simulink model "main"  (R2024a)
settings: Solver=VariableStepAuto  StartTime=0.0  StopTime=1  MaxStep=1e-4  RelTol=1e-3
InitFcn:
  | parametros
values from neighbouring files (symbols this model uses):
  alpha_cu = 3.9 *10^-3    (= 0.0039)    [parametros.m]
  b_l = 0.1    [parametros.m]
  b_m = 1.5 * 10^-5    (= 1.5e-05)    [parametros.m]
  C_ts = 0.818    [parametros.m]
  J_l = (m*l_cm^2 + J_cm) + (m_l * l_l^2)    (= 0.0833)    [parametros.m]
  J_m = 1.4 * 10^-5    (= 1.4e-05)    [parametros.m]
  k_l = m * g * l_cm + m_l * g * l_l    (= 2.4516625)    [parametros.m]
  L_d = 6.6 * 10^-3    (= 0.0066)    [parametros.m]
  L_ls = 0.8 * 10^-3    (= 0.0008)    [parametros.m]
  L_q = 5.8 * 10^-3    (= 0.0058)    [parametros.m]
  lambda_m = 0.016    [parametros.m]
  P_p = 3    [parametros.m]
  r = 120    [parametros.m]
  R_s_40 = 1.02    [parametros.m]
  R_ts_amb = 146.7    [parametros.m]
  Temp_s_ref = 40    [parametros.m]
(part 1 of 3)
settings Model: Creator=Usuario  LastModifiedBy=Usuario
settings RTWCC: GPUComputeCapability=3.5

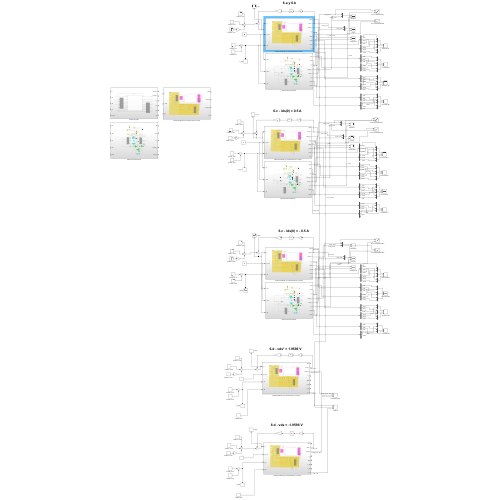
[thumbnail: Simulink's stored preview of the top-level diagram]
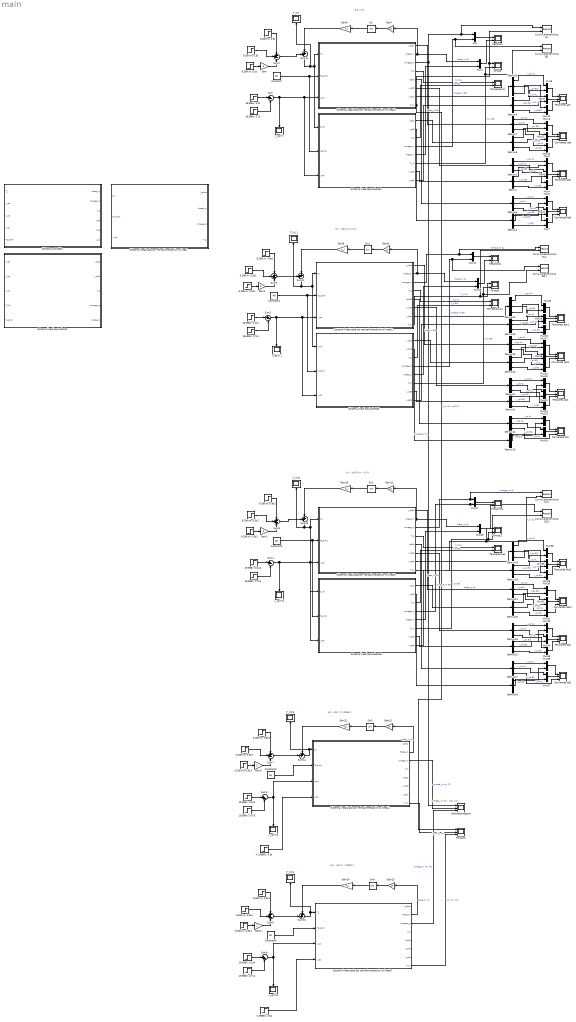
== system main ==
  note: omega_m NL - vds = 0
  note: 6.a y 6.b
  note: 6.c - ids(0) = 0.5 A
  note: 6.c - ids(0) = - 0.5 A
  note: 6.d - vds = -1.9596 V
  note: 6.d - vds* = 1.9596 V
  "+1.9596V, 0.5s" : Step  Time=.5  After=1.9596  SampleTime=0
  "-1.9596V, 0.5s" : Step  Time=.5  After=-1.9596  SampleTime=0
  19.596V, 0.1s{,1..4} (5 alike) : Step  Time=.1  After=19.596  SampleTime=0
  19.596V, 0.7s{,1..4} (5 alike) : Step  Time=.7  After=19.596  SampleTime=0
  6.28N.m, 0.3s{,1..4} (5 alike) : Step  Time=0.3  After=6.28  SampleTime=0
  6.28N.m, 0.5s{,1..4} (5 alike) : Step  Time=.5  After=6.28  SampleTime=0
  6.28N.m, 0.9s{,1..4} (5 alike) : Step  Time=.9  After=6.28  SampleTime=0
  Constant{,1..4} (5 alike) : Constant  Value=40
  Corrientes abc : Scope  NumInputPorts=3
  Corrientes abc1 : Scope  NumInputPorts=3
  Corrientes abc2 : Scope  NumInputPorts=3
  Corrientes qd0 : Scope  NumInputPorts=3
  Corrientes qd1 : Scope  NumInputPorts=3
  Corrientes qd2 : Scope  NumInputPorts=3
  Curva característica EQ : Record  FileSettingsInternal="{\"entries\":[{\"content\":{\"excelSettings\":{\"content\":{},\"type\":\"Streamout.ExcelSettings\"}},\"type\":\"Streamout.FileSettingStorage\",\"uuid\":\"\"}],\"packageUris\":[\"http:\\/\\/schema.mathworks.com\\/mf0\\/streamout_blocks\\/R2020a\"],\"version\":\"1.0\"}"  Layout=[1 1]  SignalsInternal="{\"entries\":[{\"content\":{},\"type\":\"RecordBlkView.InputSignals\",\"uuid\":\"\"}],\"packageUris\":[\"http:\\/\\/schema.mathworks.com\\/mf0\\/streamout_blocks\\/R2020a\"],\"version\":\"1.0\"}"  VisualizationBindings="{\"xyplotplugin\":{\"info\":[{\"series\":[{\"bindingParametersList\":[{\"parameter\":\"X-Axis\",\"signalID\":24,\"signalName\":\"omega_m EQ\"},{\"parameter\":\"Y-Axis\",\"signalID\":27,\"signalName\":\"T_m EQ\"}],\"seriesID\":0}],\"subplotID\":1}]}}"  CompatibilityTag=XY
  Curva característica EQ1 : Record  FileSettingsInternal="{\"entries\":[{\"content\":{\"excelSettings\":{\"content\":{},\"type\":\"Streamout.ExcelSettings\"}},\"type\":\"Streamout.FileSettingStorage\",\"uuid\":\"\"}],\"packageUris\":[\"http:\\/\\/schema.mathworks.com\\/mf0\\/streamout_blocks\\/R2020a\"],\"version\":\"1.0\"}"  Layout=[1 1]  SignalsInternal="{\"entries\":[{\"content\":{},\"type\":\"RecordBlkView.InputSignals\",\"uuid\":\"\"}],\"packageUris\":[\"http:\\/\\/schema.mathworks.com\\/mf0\\/streamout_blocks\\/R2020a\"],\"version\":\"1.0\"}"  VisualizationBindings="{\"xyplotplugin\":{\"info\":[{\"series\":[{\"bindingParametersList\":[{\"parameter\":\"X-Axis\",\"signalID\":40,\"signalName\":\"omega_m EQ\"},{\"parameter\":\"Y-Axis\",\"signalID\":43,\"signalName\":\"T_m EQ\"}],\"seriesID\":0}],\"subplotID\":1}]}}"  CompatibilityTag=XY
  Curva característica EQ2 : Record  FileSettingsInternal="{\"entries\":[{\"content\":{\"excelSettings\":{\"content\":{},\"type\":\"Streamout.ExcelSettings\"}},\"type\":\"Streamout.FileSettingStorage\",\"uuid\":\"\"}],\"packageUris\":[\"http:\\/\\/schema.mathworks.com\\/mf0\\/streamout_blocks\\/R2020a\"],\"version\":\"1.0\"}"  Layout=[1 1]  SignalsInternal="{\"entries\":[{\"content\":{},\"type\":\"RecordBlkView.InputSignals\",\"uuid\":\"\"}],\"packageUris\":[\"http:\\/\\/schema.mathworks.com\\/mf0\\/streamout_blocks\\/R2020a\"],\"version\":\"1.0\"}"  VisualizationBindings="{\"xyplotplugin\":{\"info\":[{\"series\":[{\"bindingParametersList\":[{\"parameter\":\"X-Axis\",\"signalID\":48,\"signalName\":\"omega_m EQ\"},{\"parameter\":\"Y-Axis\",\"signalID\":51,\"signalName\":\"T_m EQ\"}],\"seriesID\":0}],\"subplotID\":1}]}}"  CompatibilityTag=XY
  Curva característica NL : Record  FileSettingsInternal="{\"entries\":[{\"content\":{\"excelSettings\":{\"content\":{},\"type\":\"Streamout.ExcelSettings\"}},\"type\":\"Streamout.FileSettingStorage\",\"uuid\":\"\"}],\"packageUris\":[\"http:\\/\\/schema.mathworks.com\\/mf0\\/streamout_blocks\\/R2020a\"],\"version\":\"1.0\"}"  Layout=[1 1]  SignalsInternal="{\"entries\":[{\"content\":{},\"type\":\"RecordBlkView.InputSignals\",\"uuid\":\"\"}],\"packageUris\":[\"http:\\/\\/schema.mathworks.com\\/mf0\\/streamout_blocks\\/R2020a\"],\"version\":\"1.0\"}"  VisualizationBindings="{\"xyplotplugin\":{\"info\":[{\"series\":[{\"bindingParametersList\":[{\"parameter\":\"X-Axis\",\"signalID\":32,\"signalName\":\"omega_m NL\"},{\"parameter\":\"Y-Axis\",\"signalID\":35,\"signalName\":\"T_m NL - Vds= 0\"}],\"seriesID\":0}],\"subplotID\":1}]}}"  CompatibilityTag=XY
  Curva característica NL1 : Record  FileSettingsInternal="{\"entries\":[{\"content\":{\"excelSettings\":{\"content\":{},\"type\":\"Streamout.ExcelSettings\"}},\"type\":\"Streamout.FileSettingStorage\",\"uuid\":\"\"}],\"packageUris\":[\"http:\\/\\/schema.mathworks.com\\/mf0\\/streamout_blocks\\/R2020a\"],\"version\":\"1.0\"}"  Layout=[1 1]  SignalsInternal="{\"entries\":[{\"content\":{},\"type\":\"RecordBlkView.InputSignals\",\"uuid\":\"\"}],\"packageUris\":[\"http:\\/\\/schema.mathworks.com\\/mf0\\/streamout_blocks\\/R2020a\"],\"version\":\"1.0\"}"  VisualizationBindings="{\"xyplotplugin\":{\"info\":[{\"series\":[{\"bindingParametersList\":[{\"parameter\":\"X-Axis\",\"signalID\":16,\"signalName\":\"omega_m NL\"},{\"parameter\":\"Y-Axis\",\"signalID\":19,\"signalName\":\"T_m NL\"}],\"seriesID\":0}],\"subplotID\":1}]}}"  CompatibilityTag=XY
  Curva característica NL2 : Record  FileSettingsInternal="{\"entries\":[{\"content\":{\"excelSettings\":{\"content\":{},\"type\":\"Streamout.ExcelSettings\"}},\"type\":\"Streamout.FileSettingStorage\",\"uuid\":\"\"}],\"packageUris\":[\"http:\\/\\/schema.mathworks.com\\/mf0\\/streamout_blocks\\/R2020a\"],\"version\":\"1.0\"}"  Layout=[1 1]  SignalsInternal="{\"entries\":[{\"content\":{},\"type\":\"RecordBlkView.InputSignals\",\"uuid\":\"\"}],\"packageUris\":[\"http:\\/\\/schema.mathworks.com\\/mf0\\/streamout_blocks\\/R2020a\"],\"version\":\"1.0\"}"  VisualizationBindings="{\"xyplotplugin\":{\"info\":[{\"series\":[{\"bindingParametersList\":[{\"parameter\":\"X-Axis\",\"signalID\":8,\"signalName\":\"omega_m NL\"},{\"parameter\":\"Y-Axis\",\"signalID\":11,\"signalName\":\"T_m NL\"}],\"seriesID\":0}],\"subplotID\":1}]}}"  CompatibilityTag=XY
  Demux{,1..23} (24 alike) : Demux  Outputs=3
  Gain{,1..4} (5 alike) : Gain  Gain=2
  Gain{6,8,10,12,14} (5 alike) : Gain  Gain=k_l
  Gain{7,9,11,13,15} (5 alike) : Gain  Gain=1/r
  Mecánico : Scope  NumInputPorts=2
  Mecánico1 : Scope  NumInputPorts=2
  Mecánico2 : Scope  NumInputPorts=2
  Mux{,1..39} (40 alike) : Mux  Inputs=2
  Sin{,1..4} (5 alike) : Trigonometry
  Sistema completo : Subsystem
  Sistema lineal equivalente : Subsystem
  Sistema lineal equivalente1 : Subsystem
  Sistema lineal equivalente2 : Subsystem
  Sistema lineal equivalente3 : Subsystem
  Sistema linealizado por retroalimentación no lineal : Subsystem
  Sistema linealizado por retroalimentación no lineal1 : Subsystem
  Sistema linealizado por retroalimentación no lineal2 : Subsystem
  Sistema linealizado por retroalimentación no lineal3 : Subsystem
  Sistema linealizado por retroalimentación no lineal4 : Subsystem
  Sistema linealizado por retroalimentación no lineal5 : Subsystem
  Sum{,2,4,6,8} (5 alike) : Sum  Inputs=|+-
  Sum{1,3,5,7,9} (5 alike) : Sum  Inputs=++-
  Sum{11..15} (5 alike) : Sum  Inputs=++|
  T_l(t){,1..4} (5 alike) : Scope
  Temperatura : Scope  NumInputPorts=2
  Temperatura1 : Scope  NumInputPorts=2
  Temperatura2 : Scope  NumInputPorts=2
  Tensiones abc : Scope  NumInputPorts=3
  Tensiones abc1 : Scope  NumInputPorts=3
  Tensiones abc2 : Scope  NumInputPorts=3
  Tensiones qd0 : Scope  NumInputPorts=3
  Tensiones qd1 : Scope  NumInputPorts=3
  Tensiones qd2 : Scope  NumInputPorts=3
  Torque : Scope  NumInputPorts=2
  Torque 5 : Scope  NumInputPorts=3
  Torque1 : Scope  NumInputPorts=2
  Torque2 : Scope  NumInputPorts=2
  Velocidad angular : Scope  NumInputPorts=3
  v_qs(t){,1..4} (5 alike) : Scope
  wires:
  Sistema linealizado por retroalimentación no lineal1/2(theta_m) -> Gain7/1, Mux1/1  "theta_m NL"
  Sistema linealizado por retroalimentación no lineal1/3(omega_m) -> Velocidad angular/1, Curva característica NL/1, Mux/1  "omega_m NL"
  Sistema lineal equivalente1/5(theta_m) -> Mux1/2  "theta_m EQ"
  Sistema lineal equivalente1/4(omega_m) -> Curva característica EQ/1, Mux/2  "omega_m EQ"
  "19.596V, 0.1s"/1 -> Sum/1
  "19.596V, 0.7s"/1 -> Sum/2
  Sum/1 -> Sistema lineal equivalente1/3(v_qs), Sistema linealizado por retroalimentación no lineal1/3(v_qs), v_qs(t)/1
  "6.28N.m, 0.5s"/1 -> Gain/1
  Gain/1 -> Sum1/3
  "6.28N.m, 0.3s"/1 -> Sum1/2
  "6.28N.m, 0.9s"/1 -> Sum1/1
  Sum1/1 -> Sum11/1
  Constant/1 -> Sistema lineal equivalente1/2(T_amb), Sistema linealizado por retroalimentación no lineal1/2(Tº_amb)
  Mux/1 -> Mecánico/1
  Mux1/1 -> Mecánico/2
  Sistema lineal equivalente1/6(T_m) -> Curva característica EQ/2, Torque/2  "T_m EQ"
  Sistema lineal equivalente1/3(T_s) -> Temperatura/2  "T_s EQ"
  Sistema linealizado por retroalimentación no lineal1/4(T_s) -> Temperatura/1  "T_s NL"
  Sistema lineal equivalente1/7(v_qd0) -> Demux/1
  Demux1/1 -> Mux2/1  "v_qs NL"
  Sistema linealizado por retroalimentación no lineal1/6(v_qd0) -> Demux1/1
  Demux1/2 -> Mux3/1  "v_ds NL"
  Demux/2 -> Mux3/2  "v_ds EQ"
  Demux1/3 -> Mux4/1  "v_0 NL"
  Demux/3 -> Mux4/2  "v_0 EQ"
  Mux2/1 -> Tensiones qd0/1
  Mux3/1 -> Tensiones qd0/2
  Mux4/1 -> Tensiones qd0/3
  Demux3/3 -> Mux7/1  "i_0s NL"
  Demux2/1 -> Mux5/2  "i_qs EQ"
  Mux6/1 -> Corrientes qd0/2
  Mux5/1 -> Corrientes qd0/1
  Mux7/1 -> Corrientes qd0/3
  Demux3/2 -> Mux6/1  "i_ds NL"
  Demux2/2 -> Mux6/2  "i_ds EQ"
  Demux3/1 -> Mux5/1  "i_qs NL"
  Demux2/3 -> Mux7/2  "i_0 EQ"
  Sistema lineal equivalente1/2(i_qd0) -> Demux2/1
  Sistema linealizado por retroalimentación no lineal1/5(iqd0s) -> Demux3/1
  Demux5/3 -> Mux10/1  "v_cs NL"
  Demux4/3 -> Mux10/2  "v_cs EQ"
  Demux6/3 -> Mux13/2  "i_cs EQ"
  Demux7/1 -> Mux11/1  "i_as NL"
  Demux7/2 -> Mux12/1  "i_bs NL"
  Demux6/2 -> Mux12/2  "i_bs EQ"
  Mux13/1 -> Corrientes abc/3
  Demux7/3 -> Mux13/1  "i_cs NL"
  Demux4/1 -> Mux8/2  "v_as EQ"
  Demux6/1 -> Mux11/2  "i_as EQ"
  Mux12/1 -> Corrientes abc/2
  Mux9/1 -> Tensiones abc/2
  Demux5/2 -> Mux9/1  "v_bs NL"
  Mux10/1 -> Tensiones abc/3
  Mux8/1 -> Tensiones abc/1
  Demux4/2 -> Mux9/2  "v_bs EQ"
  Demux5/1 -> Mux8/1  "v_as NL"
  Sistema linealizado por retroalimentación no lineal1/7(v_abc) -> Demux5/1
  Sistema lineal equivalente1/8(v_abc) -> Demux4/1
  Mux11/1 -> Corrientes abc/1
  Sistema linealizado por retroalimentación no lineal1/1(i_abcs) -> Demux7/1
  Sistema lineal equivalente1/1(i_abc) -> Demux6/1
  Sistema linealizado por retroalimentación no lineal1/8(T_m) -> Curva característica NL/2, Torque/1, Torque 5/1  "T_m NL - Vds= 0"
  Sistema lineal equivalente2/7(v_qd0) -> Demux8/1
  Demux9/3 -> Mux22/1  "v_0 NL"
  Mux22/1 -> Tensiones qd1/3
  Sistema lineal equivalente2/8(v_abc) -> Demux12/1
  Sistema lineal equivalente2/4(omega_m) -> Curva característica EQ1/1, Mux14/2  "omega_m EQ"
  Demux8/3 -> Mux22/2  "v_0 EQ"
  Sistema lineal equivalente2/5(theta_m) -> Mux15/2  "theta_m EQ"
  Sistema linealizado por retroalimentación no lineal2/3(omega_m) -> Curva característica NL1/1, Mux14/1  "omega_m NL"
  Demux11/1 -> Mux23/1  "i_qs NL"
  Demux11/2 -> Mux24/1  "i_ds NL"
  Demux8/1 -> Mux20/2  "v_qs EQ"
  Demux11/3 -> Corrientes qd1/3  "i_0s NL"
  Mux25/1 -> Tensiones abc1/1
  Demux13/3 -> Mux16/1  "v_cs NL"
  Demux12/2 -> Mux26/2  "v_bs EQ"
  Mux16/1 -> Tensiones abc1/3
  Demux10/1 -> Mux23/2  "i_qs EQ"
  Mux18/1 -> Corrientes abc1/2
  Demux14/2 -> Mux18/2  "i_bs EQ"
  Demux15/3 -> Mux19/1  "i_cs NL"
  Demux14/1 -> Mux17/2  "i_as EQ"
  Mux19/1 -> Corrientes abc1/3
  Mux14/1 -> Mecánico1/1
  Demux10/2 -> Mux24/2  "i_ds EQ"
  Demux14/3 -> Mux19/2  "i_cs EQ"
  Sistema linealizado por retroalimentación no lineal2/7(v_abc) -> Demux13/1
  Sistema linealizado por retroalimentación no lineal2/8(T_m) -> Curva característica NL1/2, Torque1/1  "T_m NL"
  Mux15/1 -> Mecánico1/2
  Mux21/1 -> Tensiones qd1/2
  Sistema lineal equivalente2/2(i_qd0) -> Demux10/1
  Demux12/3 -> Mux16/2  "v_cs EQ"
  "19.596V, 0.7s1"/1 -> Sum2/2
  "19.596V, 0.1s1"/1 -> Sum2/1
  "6.28N.m, 0.3s1"/1 -> Sum3/2
  "6.28N.m, 0.5s1"/1 -> Gain1/1
  "6.28N.m, 0.9s1"/1 -> Sum3/1
  Mux20/1 -> Tensiones qd1/1
  Sistema linealizado por retroalimentación no lineal2/1(i_abcs) -> Demux15/1
  Demux13/2 -> Mux26/1  "v_bs NL"
  Constant1/1 -> Sistema lineal equivalente2/2(T_amb), Sistema linealizado por retroalimentación no lineal2/2(Tº_amb)
  Demux15/2 -> Mux18/1  "i_bs NL"
  Sistema linealizado por retroalimentación no lineal2/4(T_s) -> Temperatura1/1  "T_s NL"
  Mux24/1 -> Corrientes qd1/2
  Sistema lineal equivalente2/1(i_abc) -> Demux14/1
  Mux17/1 -> Corrientes abc1/1
  Mux23/1 -> Corrientes qd1/1
  Gain1/1 -> Sum3/3
  Sistema linealizado por retroalimentación no lineal2/5(iqd0s) -> Demux11/1
  Demux12/1 -> Mux25/2  "v_as EQ"
  Demux9/2 -> Mux21/1  "v_ds NL"
  Demux13/1 -> Mux25/1  "v_as NL"
  Sistema lineal equivalente2/3(T_s) -> Temperatura1/2  "T_s EQ"
  Sum2/1 -> Sistema lineal equivalente2/3(v_qs), Sistema linealizado por retroalimentación no lineal2/3(v_qs), v_qs(t)1/1
  Sum3/1 -> Sum12/1
  Sistema linealizado por retroalimentación no lineal2/6(v_qd0) -> Demux9/1
  Sistema lineal equivalente2/6(T_m) -> Curva característica EQ1/2, Torque1/2  "T_m EQ"
  Demux8/2 -> Mux21/2  "v_ds EQ"
  Mux26/1 -> Tensiones abc1/2
  Demux9/1 -> Mux20/1  "v_qs NL"
  Demux15/1 -> Mux17/1  "i_as NL"
  Sistema lineal equivalente3/6(T_m) -> Curva característica EQ2/2, Torque2/2  "T_m EQ"
  Sistema linealizado por retroalimentación no lineal3/6(v_qd0) -> Demux23/1
  Demux22/2 -> Mux34/2  "v_ds EQ"
  Sum5/1 -> Sum13/1
  Sum4/1 -> Sistema lineal equivalente3/3(v_qs), Sistema linealizado por retroalimentación no lineal3/3(v_qs), v_qs(t)2/1
  Demux19/1 -> Mux38/1  "v_as NL"
  Sistema lineal equivalente3/3(T_s) -> Temperatura2/2  "T_s EQ"
  Gain2/1 -> Sum5/3
  Mux36/1 -> Corrientes qd2/1
  Sistema lineal equivalente3/1(i_abc) -> Demux20/1
  Mux37/1 -> Corrientes qd2/2
  Sistema linealizado por retroalimentación no lineal3/8(T_m) -> Curva característica NL2/2, Torque2/1  "T_m NL"
  Mux28/1 -> Mecánico2/2
  Mux33/1 -> Tensiones qd2/1
  "6.28N.m, 0.9s2"/1 -> Sum5/1
  "6.28N.m, 0.5s2"/1 -> Gain2/1
  "19.596V, 0.7s2"/1 -> Sum4/2
  Mux32/1 -> Corrientes abc2/3
  Demux20/2 -> Mux31/2  "i_bs EQ"
  Mux34/1 -> Tensiones qd2/2
  Mux29/1 -> Tensiones abc2/3
  Mux38/1 -> Tensiones abc2/1
  Demux17/2 -> Mux37/1  "i_ds NL"
  Sistema linealizado por retroalimentación no lineal3/5(iqd0s) -> Demux17/1
  Demux22/1 -> Mux33/2  "v_qs EQ"
  Demux18/1 -> Mux38/2  "v_as EQ"
  Demux19/3 -> Mux29/1  "v_cs NL"
  Demux18/2 -> Mux39/2  "v_bs EQ"
  Demux17/1 -> Mux36/1  "i_qs NL"
  Sistema linealizado por retroalimentación no lineal3/3(omega_m) -> Curva característica NL2/1, Mux27/1  "omega_m NL"
  Sistema linealizado por retroalimentación no lineal3/4(T_s) -> Temperatura2/1  "T_s NL"
  Sistema linealizado por retroalimentación no lineal3/7(v_abc) -> Demux19/1
  Demux16/2 -> Mux37/2  "i_ds EQ"
  "19.596V, 0.1s2"/1 -> Sum4/1
  Constant2/1 -> Sistema lineal equivalente3/2(T_amb), Sistema linealizado por retroalimentación no lineal3/2(Tº_amb)
  Demux18/3 -> Mux29/2  "v_cs EQ"
  Demux20/1 -> Mux30/2  "i_as EQ"
  "6.28N.m, 0.3s2"/1 -> Sum5/2
  Demux22/3 -> Mux35/2  "v_0 EQ"
  Demux21/3 -> Mux32/1  "i_cs NL"
  Sistema lineal equivalente3/4(omega_m) -> Curva característica EQ2/1, Mux27/2  "omega_m EQ"
  Demux23/2 -> Mux34/1  "v_ds NL"
  Sistema lineal equivalente3/8(v_abc) -> Demux18/1
  Demux20/3 -> Mux32/2  "i_cs EQ"
  Mux31/1 -> Corrientes abc2/2
  Sistema linealizado por retroalimentación no lineal3/2(theta_m) -> Gain11/1, Mux28/1  "theta_m NL"
  Mux30/1 -> Corrientes abc2/1
  Mux39/1 -> Tensiones abc2/2
  Mux35/1 -> Tensiones qd2/3
  Sistema lineal equivalente3/2(i_qd0) -> Demux16/1
  Demux23/3 -> Mux35/1  "v_0 NL"
  Mux27/1 -> Mecánico2/1
  Sistema lineal equivalente3/5(theta_m) -> Mux28/2  "theta_m EQ"
  Demux16/1 -> Mux36/2  "i_qs EQ"
  Demux19/2 -> Mux39/1  "v_bs NL"
  Demux23/1 -> Mux33/1  "v_qs NL"
  Sistema lineal equivalente3/7(v_qd0) -> Demux22/1
  Demux21/1 -> Mux30/1  "i_as NL"
  Demux21/2 -> Mux31/1  "i_bs NL"
  Demux17/3 -> Corrientes qd2/3  "i_0s NL"
  "19.596V, 0.7s3"/1 -> Sum6/2
  Gain3/1 -> Sum7/3
  Sum6/1 -> Sistema linealizado por retroalimentación no lineal4/3(v_qs), v_qs(t)3/1
  "6.28N.m, 0.9s3"/1 -> Sum7/1
  "6.28N.m, 0.5s3"/1 -> Gain3/1
  Sum7/1 -> Sum14/2
  "6.28N.m, 0.3s3"/1 -> Sum7/2
  "19.596V, 0.1s3"/1 -> Sum6/1
  Constant3/1 -> Sistema linealizado por retroalimentación no lineal4/2(Tº_amb)
  Constant4/1 -> Sistema linealizado por retroalimentación no lineal5/2(Tº_amb)
  "19.596V, 0.1s4"/1 -> Sum8/1
  Sum9/1 -> Sum15/2
  "6.28N.m, 0.3s4"/1 -> Sum9/2
  "6.28N.m, 0.9s4"/1 -> Sum9/1
  Sum8/1 -> Sistema linealizado por retroalimentación no lineal5/3(v_qs), v_qs(t)4/1
  Gain4/1 -> Sum9/3
  "6.28N.m, 0.5s4"/1 -> Gain4/1
  "19.596V, 0.7s4"/1 -> Sum8/2
  "-1.9596V, 0.5s"/1 -> Sistema linealizado por retroalimentación no lineal5/4(v_ds)
  "+1.9596V, 0.5s"/1 -> Sistema linealizado por retroalimentación no lineal4/4(v_ds)
  Demux/1 -> Mux2/2  "v_qs EQ"
  Sistema linealizado por retroalimentación no lineal4/3(omega_m) -> Velocidad angular/2  "omega_m NL - FF"
  Sistema linealizado por retroalimentación no lineal5/3(omega_m) -> Velocidad angular/3  "omega_m NL - FW"
  Sistema linealizado por retroalimentación no lineal5/8(T_m) -> Torque 5/3  "T_m NL - FW"
  Sistema linealizado por retroalimentación no lineal4/8(T_m) -> Torque 5/2  "T_m NL - FF"
  Gain7/1 -> Sin/1
  Sin/1 -> Gain6/1
  Gain6/1 -> Sum11/2
  Sum11/1 -> Sistema linealizado por retroalimentación no lineal1/1(T_l), Sistema lineal equivalente1/1(T_l(t)), T_l(t)/1
  Sin1/1 -> Gain8/1
  Gain9/1 -> Sin1/1
  Sistema linealizado por retroalimentación no lineal2/2(theta_m) -> Gain9/1, Mux15/1  "theta_m NL"
  Gain8/1 -> Sum12/2
  Sum12/1 -> Sistema lineal equivalente2/1(T_l(t)), Sistema linealizado por retroalimentación no lineal2/1(T_l), T_l(t)1/1
  Sin2/1 -> Gain10/1
  Gain11/1 -> Sin2/1
  Sistema linealizado por retroalimentación no lineal3/1(i_abcs) -> Demux21/1  "theta_m NL"
  Sum13/1 -> Sistema lineal equivalente3/1(T_l(t)), Sistema linealizado por retroalimentación no lineal3/1(T_l), T_l(t)2/1
  Gain10/1 -> Sum13/2
  Gain13/1 -> Sin3/1
  Sin3/1 -> Gain12/1
  Gain12/1 -> Sum14/1
  Sum14/1 -> Sistema linealizado por retroalimentación no lineal4/1(T_l), T_l(t)3/1
  Sistema linealizado por retroalimentación no lineal4/2(theta_m) -> Gain13/1  "theta_m NL"
  Gain15/1 -> Sin4/1
  Sin4/1 -> Gain14/1
  Gain14/1 -> Sum15/1
  Sum15/1 -> Sistema linealizado por retroalimentación no lineal5/1(T_l), T_l(t)4/1
  Sistema linealizado por retroalimentación no lineal5/2(theta_m) -> Gain15/1  "theta_m NL"

== system main/Sistema completo ==
  T_l : Inport
  v_as : Inport  Port=2
  v_bs : Inport  Port=3
  v_cs : Inport  Port=4
  Tº_amb : Inport  Port=5
  Gain : Gain  Gain=P_p
  Subsistema físico no lineal : Subsystem
  TD_PARK : MATLAB Function  TreatAsAtomicUnit=on
  TI_PARK : MATLAB Function  TreatAsAtomicUnit=on
  theta_m : Outport
  omega_m : Outport  Port=2
  T_s : Outport  Port=3
  i_as : Outport  Port=4
  i_bs : Outport  Port=5
  i_cs : Outport  Port=6
  wires:
  Subsistema físico no lineal/1(theta_m) -> theta_m/1, Gain/1
  TI_PARK/2(fbs) -> i_bs/1
  v_cs/1 -> TD_PARK/3(fcs)
  v_as/1 -> TD_PARK/1(fas)
  TI_PARK/3(fcs) -> i_cs/1
  v_bs/1 -> TD_PARK/2(fbs)
  TI_PARK/1(fas) -> i_as/1
  T_l/1 -> Subsistema físico no lineal/1(T_l)
  TD_PARK/1(fqs) -> Subsistema físico no lineal/2(v_qs^r)
  TD_PARK/2(fds) -> Subsistema físico no lineal/3(v_ds^r)
  TD_PARK/3(f0s) -> Subsistema físico no lineal/4(v_0s^r)
  Tº_amb/1 -> Subsistema físico no lineal/5(Tº_amb)
  Subsistema físico no lineal/2(omega_m) -> omega_m/1
  Subsistema físico no lineal/3(T_s) -> T_s/1
  Subsistema físico no lineal/4(i_qs^r) -> TI_PARK/1(fqs)
  Subsistema físico no lineal/5(i_ds^r) -> TI_PARK/2(fds)
  Subsistema físico no lineal/6(i_0s^r) -> TI_PARK/3(f0s)
  Gain/1 -> TI_PARK/4(theta_r), TD_PARK/4(theta_r)

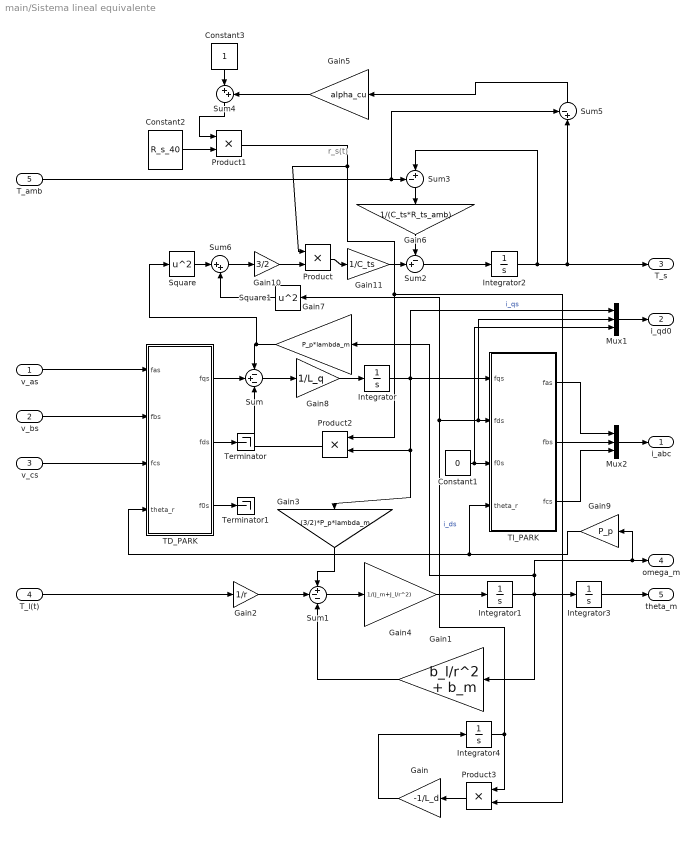
== system main/Sistema lineal equivalente ==
  note: r_s(t)
  v_as : Inport
  v_bs : Inport  Port=2
  v_cs : Inport  Port=3
  T_l(t) : Inport  Port=4
  T_amb : Inport  Port=5
  Constant1 : Constant  Value=0
  Constant2 : Constant  Value=R_s_40
  Constant3 : Constant
  Gain : Gain  Gain=-1/L_d
  Gain1 : Gain  Gain=b_l/r^2 + b_m
  Gain10 : Gain  Gain=3/2
  Gain11 : Gain  Gain=1/C_ts
  Gain2 : Gain  Gain=1/r
  Gain3 : Gain  Gain=(3/2)*P_p*lambda_m
  Gain4 : Gain  Gain=1/(J_m+J_l/r^2)
  Gain5 : Gain  Gain=alpha_cu
  Gain6 : Gain  Gain=1/(C_ts*R_ts_amb)
  Gain7 : Gain  Gain=P_p*lambda_m
  Gain8 : Gain  Gain=1/L_q
  Gain9 : Gain  Gain=P_p
  Integrator{,1..4} (5 alike) : Integrator
  Mux1 : Mux  Inputs=3
  Mux2 : Mux  Inputs=3
  Product{,1..3} (4 alike) : Product
  Square : Math  Operator=square
  Square1 : Math  Operator=square
  Sum : Sum  Inputs=-+-
  Sum1 : Sum  Inputs=+--
  Sum2 : Sum  Inputs=-+|
  Sum3 : Sum  Inputs=-+|
  Sum4 : Sum  Inputs=|++
  Sum5 : Sum  Inputs=-+|
  Sum6 : Sum  Inputs=|++
  TD_PARK : MATLAB Function  TreatAsAtomicUnit=on
  TI_PARK : MATLAB Function  TreatAsAtomicUnit=on
  Terminator : Terminator
  Terminator1 : Terminator
  i_abc : Outport
  i_qd0 : Outport  Port=2
  T_s : Outport  Port=3
  omega_m : Outport  Port=4
  theta_m : Outport  Port=5
  wires:
  Integrator/1 -> Mux1/1, TI_PARK/1(fqs), Product2/2, Gain3/1  "i_qs"
  Product2/1 -> Sum/3
  TD_PARK/1(fqs) -> Sum/2
  Sum/1 -> Gain8/1
  Integrator1/1 -> Gain7/1, Gain9/1, omega_m/1, Integrator3/1, Gain1/1
  Sum1/1 -> Gain4/1
  Gain1/1 -> Sum1/3
  Gain4/1 -> Integrator1/1
  Integrator4/1 -> Product3/1, Mux1/2, TI_PARK/2(fds), Square1/1  "i_ds"
  Constant1/1 -> TI_PARK/3(f0s), Mux1/3
  TI_PARK/1(fas) -> Mux2/1
  TI_PARK/2(fbs) -> Mux2/2
  TI_PARK/3(fcs) -> Mux2/3
  Gain2/1 -> Sum1/2
  Sum3/1 -> Gain6/1
  Gain6/1 -> Sum2/1
  Sum2/1 -> Integrator2/1
  TD_PARK/2(fds) -> Terminator/1
  TD_PARK/3(f0s) -> Terminator1/1
  Integrator3/1 -> theta_m/1
  v_as/1 -> TD_PARK/1(fas)
  v_bs/1 -> TD_PARK/2(fbs)
  v_cs/1 -> TD_PARK/3(fcs)
  Gain9/1 -> TI_PARK/4(theta_r), TD_PARK/4(theta_r)
  T_amb/1 -> Sum5/1, Sum3/1
  T_l(t)/1 -> Gain2/1
  Mux2/1 -> i_abc/1
  Mux1/1 -> i_qd0/1
  Integrator2/1 -> Sum5/2, T_s/1, Sum3/2
  Gain8/1 -> Integrator/1
  Gain7/1 -> Square/1, Sum/1
  Gain3/1 -> Sum1/1
  Gain10/1 -> Product/2
  Product/1 -> Gain11/1
  Gain11/1 -> Sum2/2
  Sum5/1 -> Gain5/1
  Gain5/1 -> Sum4/2
  Constant3/1 -> Sum4/1
  Constant2/1 -> Product1/2
  Sum4/1 -> Product1/1
  Product1/1 -> Product3/2, Product2/1, Product/1
  Product3/1 -> Gain/1
  Gain/1 -> Integrator4/1
  Square/1 -> Sum6/1
  Sum6/1 -> Gain10/1
  Square1/1 -> Sum6/2

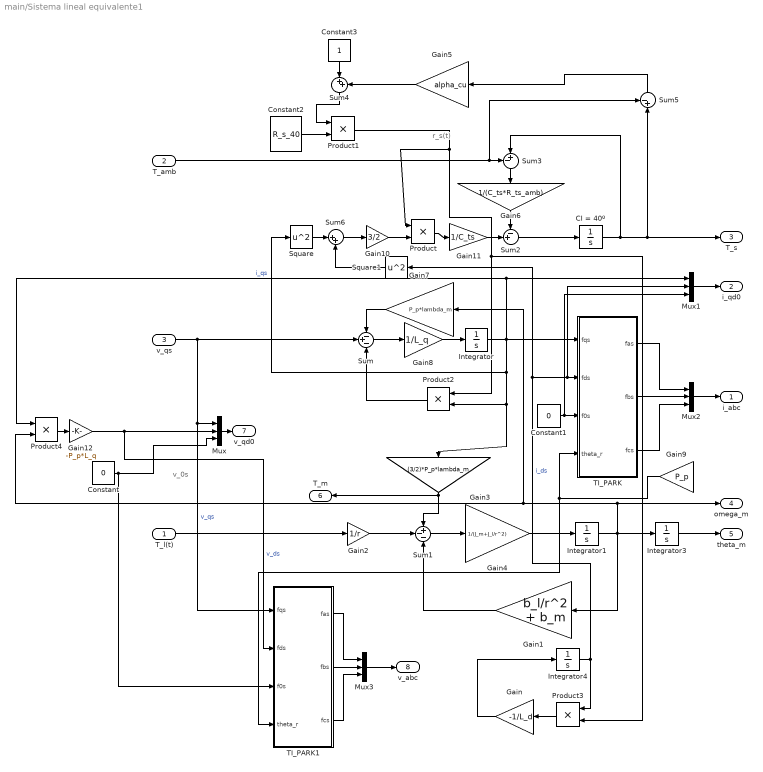
== system main/Sistema lineal equivalente1 ==
  note: v_0s
  note: r_s(t)
  T_l(t) : Inport
  T_amb : Inport  Port=2
  v_qs : Inport  Port=3
  CI = 40º : Integrator  InitialCondition=40
  Constant : Constant  Value=0
  Constant1 : Constant  Value=0
  Constant2 : Constant  Value=R_s_40
  Constant3 : Constant
  Gain : Gain  Gain=-1/L_d
  Gain1 : Gain  Gain=b_l/r^2 + b_m
  Gain10 : Gain  Gain=3/2
  Gain11 : Gain  Gain=1/C_ts
  Gain12 : Gain  Gain=-P_p*L_q
  Gain2 : Gain  Gain=1/r
  Gain3 : Gain  Gain=(3/2)*P_p*lambda_m
  Gain4 : Gain  Gain=1/(J_m+J_l/r^2)
  Gain5 : Gain  Gain=alpha_cu
  Gain6 : Gain  Gain=1/(C_ts*R_ts_amb)
  Gain7 : Gain  Gain=P_p*lambda_m
  Gain8 : Gain  Gain=1/L_q
  Gain9 : Gain  Gain=P_p
  Integrator{,1,3..4} (4 alike) : Integrator
  Mux{,1..3} (4 alike) : Mux  Inputs=3
  Product{,1..4} (5 alike) : Product
  Square : Math  Operator=square
  Square1 : Math  Operator=square
  Sum : Sum  Inputs=-+-
  Sum1 : Sum  Inputs=+--
  Sum2 : Sum  Inputs=-+|
  Sum3 : Sum  Inputs=-+|
  Sum4 : Sum  Inputs=|++
  Sum5 : Sum  Inputs=-+|
  Sum6 : Sum  Inputs=|++
  TI_PARK : MATLAB Function  TreatAsAtomicUnit=on
  TI_PARK1 : MATLAB Function  TreatAsAtomicUnit=on
  i_abc : Outport
  i_qd0 : Outport  Port=2
  T_s : Outport  Port=3
  omega_m : Outport  Port=4
  theta_m : Outport  Port=5
  T_m : Outport  Port=6
  v_qd0 : Outport  Port=7
  v_abc : Outport  Port=8
  wires:
  Integrator/1 -> Square/1, Product2/2, Gain3/1, Mux1/1, Product4/1, TI_PARK/1(fqs)  "i_qs"
  Product2/1 -> Sum/3
  v_qs/1 -> TI_PARK1/1(fqs), Mux/1, Sum/2  "v_qs"
  Sum/1 -> Gain8/1
  Integrator1/1 -> Gain7/1, Product4/2, omega_m/1, Integrator3/1, Gain1/1
  Sum1/1 -> Gain4/1
  Gain1/1 -> Sum1/3
  Gain4/1 -> Integrator1/1
  Integrator4/1 -> Product3/1, Mux1/2, TI_PARK/2(fds), Square1/1  "i_ds"
  Constant1/1 -> TI_PARK/3(f0s), Mux1/3
  TI_PARK/1(fas) -> Mux2/1
  TI_PARK/2(fbs) -> Mux2/2
  TI_PARK/3(fcs) -> Mux2/3
  Gain2/1 -> Sum1/2
  Sum3/1 -> Gain6/1
  Gain6/1 -> Sum2/1
  Sum2/1 -> CI = 40º/1
  Integrator3/1 -> theta_m/1
  Gain9/1 -> TI_PARK/4(theta_r), TI_PARK1/4(theta_r)
  T_amb/1 -> Sum5/1, Sum3/1
  T_l(t)/1 -> Gain2/1
  Mux2/1 -> i_abc/1
  Mux1/1 -> i_qd0/1
  CI = 40º/1 -> Sum5/2, T_s/1, Sum3/2
  Gain8/1 -> Integrator/1
  Gain7/1 -> Sum/1
  Gain3/1 -> T_m/1, Sum1/1
  Gain10/1 -> Product/2
  Product/1 -> Gain11/1
  Gain11/1 -> Sum2/2
  Sum5/1 -> Gain5/1
  Gain5/1 -> Sum4/2
  Constant3/1 -> Sum4/1
  Constant2/1 -> Product1/2
  Sum4/1 -> Product1/1
  Product1/1 -> Product2/1, Product3/2, Product/1
  Product3/1 -> Gain/1
  Gain/1 -> Integrator4/1
  Square/1 -> Sum6/1
  Sum6/1 -> Gain10/1
  Square1/1 -> Sum6/2
  Gain12/1 -> TI_PARK1/2(fds), Mux/2  "v_ds"
  Product4/1 -> Gain12/1
  Constant/1 -> TI_PARK1/3(f0s), Mux/3
  Mux/1 -> v_qd0/1
  TI_PARK1/1(fas) -> Mux3/1
  TI_PARK1/3(fcs) -> Mux3/3
  TI_PARK1/2(fbs) -> Mux3/2
  Mux3/1 -> v_abc/1

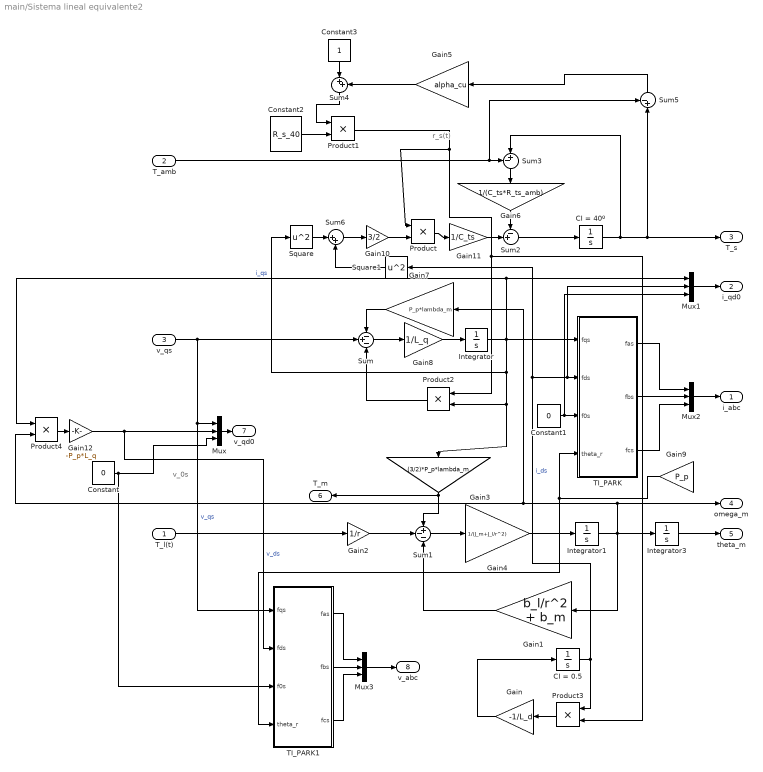
== system main/Sistema lineal equivalente2 ==
  note: v_0s
  note: r_s(t)
  T_l(t) : Inport
  T_amb : Inport  Port=2
  v_qs : Inport  Port=3
  CI = 0.5 : Integrator  InitialCondition=0.5
  CI = 40º : Integrator  InitialCondition=40
  Constant : Constant  Value=0
  Constant1 : Constant  Value=0
  Constant2 : Constant  Value=R_s_40
  Constant3 : Constant
  Gain : Gain  Gain=-1/L_d
  Gain1 : Gain  Gain=b_l/r^2 + b_m
  Gain10 : Gain  Gain=3/2
  Gain11 : Gain  Gain=1/C_ts
  Gain12 : Gain  Gain=-P_p*L_q
  Gain2 : Gain  Gain=1/r
  Gain3 : Gain  Gain=(3/2)*P_p*lambda_m
  Gain4 : Gain  Gain=1/(J_m+J_l/r^2)
  Gain5 : Gain  Gain=alpha_cu
  Gain6 : Gain  Gain=1/(C_ts*R_ts_amb)
  Gain7 : Gain  Gain=P_p*lambda_m
  Gain8 : Gain  Gain=1/L_q
  Gain9 : Gain  Gain=P_p
  Integrator : Integrator
  Integrator1 : Integrator
  Integrator3 : Integrator
  Mux{,1..3} (4 alike) : Mux  Inputs=3
  Product{,1..4} (5 alike) : Product
  Square : Math  Operator=square
  Square1 : Math  Operator=square
  Sum : Sum  Inputs=-+-
  Sum1 : Sum  Inputs=+--
  Sum2 : Sum  Inputs=-+|
  Sum3 : Sum  Inputs=-+|
  Sum4 : Sum  Inputs=|++
  Sum5 : Sum  Inputs=-+|
  Sum6 : Sum  Inputs=|++
  TI_PARK : MATLAB Function  TreatAsAtomicUnit=on
  TI_PARK1 : MATLAB Function  TreatAsAtomicUnit=on
  i_abc : Outport
  i_qd0 : Outport  Port=2
  T_s : Outport  Port=3
  omega_m : Outport  Port=4
  theta_m : Outport  Port=5
  T_m : Outport  Port=6
  v_qd0 : Outport  Port=7
  v_abc : Outport  Port=8
  wires:
  Integrator/1 -> Square/1, Product2/2, Gain3/1, Mux1/1, Product4/1, TI_PARK/1(fqs)  "i_qs"
  Product2/1 -> Sum/3
  v_qs/1 -> TI_PARK1/1(fqs), Mux/1, Sum/2  "v_qs"
  Sum/1 -> Gain8/1
  Integrator1/1 -> Gain7/1, Product4/2, omega_m/1, Integrator3/1, Gain1/1
  Sum1/1 -> Gain4/1
  Gain1/1 -> Sum1/3
  Gain4/1 -> Integrator1/1
  CI = 0.5/1 -> Product3/1, Mux1/2, TI_PARK/2(fds), Square1/1  "i_ds"
  Constant1/1 -> TI_PARK/3(f0s), Mux1/3
  TI_PARK/1(fas) -> Mux2/1
  TI_PARK/2(fbs) -> Mux2/2
  TI_PARK/3(fcs) -> Mux2/3
  Gain2/1 -> Sum1/2
  Sum3/1 -> Gain6/1
  Gain6/1 -> Sum2/1
  Sum2/1 -> CI = 40º/1
  Integrator3/1 -> theta_m/1
  Gain9/1 -> TI_PARK/4(theta_r), TI_PARK1/4(theta_r)
  T_amb/1 -> Sum5/1, Sum3/1
  T_l(t)/1 -> Gain2/1
  Mux2/1 -> i_abc/1
  Mux1/1 -> i_qd0/1
  CI = 40º/1 -> Sum5/2, T_s/1, Sum3/2
  Gain8/1 -> Integrator/1
  Gain7/1 -> Sum/1
  Gain3/1 -> T_m/1, Sum1/1
  Gain10/1 -> Product/2
  Product/1 -> Gain11/1
  Gain11/1 -> Sum2/2
  Sum5/1 -> Gain5/1
  Gain5/1 -> Sum4/2
  Constant3/1 -> Sum4/1
  Constant2/1 -> Product1/2
  Sum4/1 -> Product1/1
  Product1/1 -> Product2/1, Product3/2, Product/1
  Product3/1 -> Gain/1
  Gain/1 -> CI = 0.5/1
  Square/1 -> Sum6/1
  Sum6/1 -> Gain10/1
  Square1/1 -> Sum6/2
  Gain12/1 -> TI_PARK1/2(fds), Mux/2  "v_ds"
  Product4/1 -> Gain12/1
  Constant/1 -> TI_PARK1/3(f0s), Mux/3
  Mux/1 -> v_qd0/1
  TI_PARK1/1(fas) -> Mux3/1
  TI_PARK1/3(fcs) -> Mux3/3
  TI_PARK1/2(fbs) -> Mux3/2
  Mux3/1 -> v_abc/1

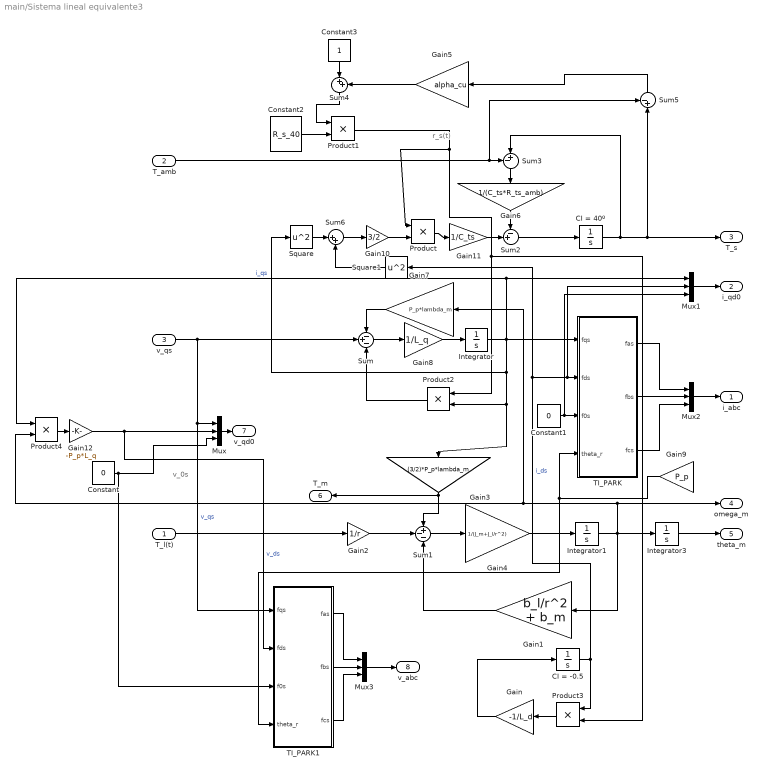
== system main/Sistema lineal equivalente3 ==
  note: v_0s
  note: r_s(t)
  T_l(t) : Inport
  T_amb : Inport  Port=2
  v_qs : Inport  Port=3
  CI = -0.5 : Integrator  InitialCondition=-0.5
  CI = 40º : Integrator  InitialCondition=40
  Constant : Constant  Value=0
  Constant1 : Constant  Value=0
  Constant2 : Constant  Value=R_s_40
  Constant3 : Constant
  Gain : Gain  Gain=-1/L_d
  Gain1 : Gain  Gain=b_l/r^2 + b_m
  Gain10 : Gain  Gain=3/2
  Gain11 : Gain  Gain=1/C_ts
  Gain12 : Gain  Gain=-P_p*L_q
  Gain2 : Gain  Gain=1/r
  Gain3 : Gain  Gain=(3/2)*P_p*lambda_m
  Gain4 : Gain  Gain=1/(J_m+J_l/r^2)
  Gain5 : Gain  Gain=alpha_cu
  Gain6 : Gain  Gain=1/(C_ts*R_ts_amb)
  Gain7 : Gain  Gain=P_p*lambda_m
  Gain8 : Gain  Gain=1/L_q
  Gain9 : Gain  Gain=P_p
  Integrator : Integrator
  Integrator1 : Integrator
  Integrator3 : Integrator
  Mux{,1..3} (4 alike) : Mux  Inputs=3
  Product{,1..4} (5 alike) : Product
  Square : Math  Operator=square
  Square1 : Math  Operator=square
  Sum : Sum  Inputs=-+-
  Sum1 : Sum  Inputs=+--
  Sum2 : Sum  Inputs=-+|
  Sum3 : Sum  Inputs=-+|
  Sum4 : Sum  Inputs=|++
  Sum5 : Sum  Inputs=-+|
  Sum6 : Sum  Inputs=|++
  TI_PARK : MATLAB Function  TreatAsAtomicUnit=on
  TI_PARK1 : MATLAB Function  TreatAsAtomicUnit=on
  i_abc : Outport
  i_qd0 : Outport  Port=2
  T_s : Outport  Port=3
  omega_m : Outport  Port=4
  theta_m : Outport  Port=5
  T_m : Outport  Port=6
  v_qd0 : Outport  Port=7
  v_abc : Outport  Port=8
  wires:
  Integrator/1 -> Square/1, Product2/2, Gain3/1, Mux1/1, Product4/1, TI_PARK/1(fqs)  "i_qs"
  Product2/1 -> Sum/3
  v_qs/1 -> TI_PARK1/1(fqs), Mux/1, Sum/2  "v_qs"
  Sum/1 -> Gain8/1
  Integrator1/1 -> Gain7/1, Product4/2, omega_m/1, Integrator3/1, Gain1/1
  Sum1/1 -> Gain4/1
  Gain1/1 -> Sum1/3
  Gain4/1 -> Integrator1/1
  CI = -0.5/1 -> Product3/1, Mux1/2, TI_PARK/2(fds), Square1/1  "i_ds"
  Constant1/1 -> TI_PARK/3(f0s), Mux1/3
  TI_PARK/1(fas) -> Mux2/1
  TI_PARK/2(fbs) -> Mux2/2
  TI_PARK/3(fcs) -> Mux2/3
  Gain2/1 -> Sum1/2
  Sum3/1 -> Gain6/1
  Gain6/1 -> Sum2/1
  Sum2/1 -> CI = 40º/1
  Integrator3/1 -> theta_m/1
  Gain9/1 -> TI_PARK/4(theta_r), TI_PARK1/4(theta_r)
  T_amb/1 -> Sum5/1, Sum3/1
  T_l(t)/1 -> Gain2/1
  Mux2/1 -> i_abc/1
  Mux1/1 -> i_qd0/1
  CI = 40º/1 -> Sum5/2, T_s/1, Sum3/2
  Gain8/1 -> Integrator/1
  Gain7/1 -> Sum/1
  Gain3/1 -> T_m/1, Sum1/1
  Gain10/1 -> Product/2
  Product/1 -> Gain11/1
  Gain11/1 -> Sum2/2
  Sum5/1 -> Gain5/1
  Gain5/1 -> Sum4/2
  Constant3/1 -> Sum4/1
  Constant2/1 -> Product1/2
  Sum4/1 -> Product1/1
  Product1/1 -> Product2/1, Product3/2, Product/1
  Product3/1 -> Gain/1
  Gain/1 -> CI = -0.5/1
  Square/1 -> Sum6/1
  Sum6/1 -> Gain10/1
  Square1/1 -> Sum6/2
  Gain12/1 -> TI_PARK1/2(fds), Mux/2  "v_ds"
  Product4/1 -> Gain12/1
  Constant/1 -> TI_PARK1/3(f0s), Mux/3
  Mux/1 -> v_qd0/1
  TI_PARK1/1(fas) -> Mux3/1
  TI_PARK1/3(fcs) -> Mux3/3
  TI_PARK1/2(fbs) -> Mux3/2
  Mux3/1 -> v_abc/1

== system main/Sistema linealizado por retroalimentación no lineal ==
  note: Entrada de perturbación
  note: Entrada de manipulación
  note: Entrada de perturbación
  note: Controlador
  note: Salida medida
  note: Controlador
  note: Sensores
  note: Salida medida
  note: Salidas medida
  note: Salida no medida.
  note: Controlador
  T_l : Inport
  Tº_amb : Inport  Port=2
  v_qs : Inport  Port=3
  Constant : Constant  Value=0
  Gain{,1..4} (5 alike) : Gain
  Gain10 : Gain  Gain=L_q
  Gain11 : Gain  Gain=-1
  Gain5 : Gain  Gain=P_p
  Gain6 : Gain  Gain=L_d
  Gain8 : Gain  Gain=P_p
  Gain9 : Gain  Gain=P_p
  Inversor: Modulador de tensión : Subsystem
  Mux : Mux  Inputs=3
  Product : Product
  Product1 : Product
  "Subsistema físico no lineal " : Subsystem
      settings: PortSchema="{\"entries\":[{\"content\":{\"sides\":[{\"content\":{\"connectorIds\":[\"In1\",\"In2\",\"In3\",\"In4\",\"In5\",\"In6\"]},\"type\":\"ConnectorPlacement.EquallySpacedRectSide\",\"uuid\":\"df16c937-5b0d-437b-9581-4e7e4443d731\"},{\"content\":{\"connectorIds\":[\"Out1\",\"Out2\",\"Out3\",\"Out4\",\"Out5\"],\"side\":\"RIGHT\"},\"type\":\"ConnectorPlacement.EquallySpacedRectSide\",\"uuid\":\"58799b56-1bb2-4861-ad63-3fa3f8181ad5\"},{\"content\":{\"connectorIds\":[\"Out6\"],\"side\":\"TOP\"},\"type\":\"ConnectorPlacement.EquallySpacedRectSide\",\"uuid\":\"9d658df7-49d2-4fa1-a84c-b158d9dac98e\"}]},\"type\":\"ConnectorPlacement.EquallySpacedConnector\",\"uuid\":\"4e139d46-6a94-417e-9cad-9c9676c83a39\"}],\"packageUris\":[\"http://schema.mathworks.com/mf0/Connector/R2020b\"],\"version\":\"1.0\"}"
  Sum : Sum  Inputs=|++
  TD_PARK : MATLAB Function  TreatAsAtomicUnit=on
  TI_PARK : MATLAB Function  TreatAsAtomicUnit=on
  Terminator1 : Terminator
  i_abcs : Outport
  theta_m : Outport  Port=2
  omega_m : Outport  Port=3
  T_s : Outport  Port=4
  wires:
  T_l/1 -> "Subsistema físico no lineal "/1(T_l)
  "Subsistema físico no lineal "/2(T_s) -> Gain1/1
  "Subsistema físico no lineal "/1(theta_m) -> Gain/1
  Tº_amb/1 -> "Subsistema físico no lineal "/6(Tº_amb)
  "Subsistema físico no lineal "/4(i_bs) -> Gain3/1
  "Subsistema físico no lineal "/5(i_cs) -> Gain4/1
  "Subsistema físico no lineal "/3(i_as) -> Gain2/1
  Gain2/1 -> TD_PARK/1(fas), Mux/1
  Gain3/1 -> TD_PARK/2(fbs), Mux/2
  Gain4/1 -> TD_PARK/3(fcs), Mux/3
  Mux/1 -> i_abcs/1
  Gain/1 -> Gain8/1, theta_m/1
  "Subsistema físico no lineal "/6(omega_m) -> Product1/1, Product/1, omega_m/1  "omega_m"
  Gain1/1 -> T_s/1
  Gain8/1 -> "Subsistema físico no lineal "/5(theta_r), TI_PARK/4(theta_r), TD_PARK/4(theta_r)  "theta_r"
  TD_PARK/1(fqs) -> Product/2  "i_qs^r"
  Product/1 -> Gain9/1
  Gain9/1 -> Gain10/1
  Gain11/1 -> TI_PARK/2(fds)
  Gain10/1 -> Gain11/1
  Constant/1 -> TI_PARK/3(f0s)
  Inversor: Modulador de tensión/1(v_as) -> "Subsistema físico no lineal "/2(v_as)
  Inversor: Modulador de tensión/2(v_bs) -> "Subsistema físico no lineal "/3(v_bs)
  Inversor: Modulador de tensión/3(v_cs) -> "Subsistema físico no lineal "/4(v_cs)
  TI_PARK/1(fas) -> Inversor: Modulador de tensión/1(v_as*)
  TI_PARK/2(fbs) -> Inversor: Modulador de tensión/2(v_bs*)
  TI_PARK/3(fcs) -> Inversor: Modulador de tensión/3(v_cs*)
  TD_PARK/2(fds) -> Product1/2
  TD_PARK/3(f0s) -> Terminator1/1
  v_qs/1 -> Sum/1
  Sum/1 -> TI_PARK/1(fqs)
  Product1/1 -> Gain5/1
  Gain5/1 -> Gain6/1
  Gain6/1 -> Sum/2

== system main/Sistema linealizado por retroalimentación no lineal1 ==
  note: Entrada de perturbación
  note: Entrada de manipulación
  note: Entrada de perturbación
  note: Controlador
  note: Salida medida
  note: Controlador
  note: Sensores
  note: Salida medida
  note: Salidas medidas
  note: Salida no medida.
  note: Controlador
  T_l : Inport
  Tº_amb : Inport  Port=2
  v_qs : Inport  Port=3
  Constant : Constant  Value=0
  Gain{,1..4} (5 alike) : Gain
  Gain10 : Gain  Gain=L_q
  Gain11 : Gain  Gain=-1
  Gain5 : Gain  Gain=P_p
  Gain6 : Gain  Gain=L_d
  Gain8 : Gain  Gain=P_p
  Gain9 : Gain  Gain=P_p
  Inversor: Modulador de tensión : Subsystem
  Mux : Mux  Inputs=3
  Mux1 : Mux  Inputs=3
  Mux2 : Mux  Inputs=3
  Product : Product
  Product1 : Product
  "Subsistema físico no lineal " : Subsystem
      settings: PortSchema="{\"entries\":[{\"content\":{\"sides\":[{\"content\":{\"connectorIds\":[\"In1\",\"In2\",\"In3\",\"In4\",\"In5\",\"In6\"]},\"type\":\"ConnectorPlacement.EquallySpacedRectSide\",\"uuid\":\"df16c937-5b0d-437b-9581-4e7e4443d731\"},{\"content\":{\"connectorIds\":[\"Out1\",\"Out2\",\"Out3\",\"Out4\",\"Out5\"],\"side\":\"RIGHT\"},\"type\":\"ConnectorPlacement.EquallySpacedRectSide\",\"uuid\":\"58799b56-1bb2-4861-ad63-3fa3f8181ad5\"},{\"content\":{\"connectorIds\":[\"Out6\",\"Out7\"],\"side\":\"TOP\"},\"type\":\"ConnectorPlacement.EquallySpacedRectSide\",\"uuid\":\"9d658df7-49d2-4fa1-a84c-b158d9dac98e\"}]},\"type\":\"ConnectorPlacement.EquallySpacedConnector\",\"uuid\":\"4e139d46-6a94-417e-9cad-9c9676c83a39\"}],\"packageUris\":[\"http://schema.mathworks.com/mf0/Connector/R2020b\"],\"version\":\"1.0\"}"
  Sum : Sum  Inputs=|++
  TD_PARK : MATLAB Function  TreatAsAtomicUnit=on
  TI_PARK : MATLAB Function  TreatAsAtomicUnit=on
  mux : Mux  Inputs=3
  i_abcs : Outport
  theta_m : Outport  Port=2
  omega_m : Outport  Port=3
  T_s : Outport  Port=4
  iqd0s : Outport  Port=5
  v_qd0 : Outport  Port=6
  v_abc : Outport  Port=7
  T_m : Outport  Port=8
  wires:
  T_l/1 -> "Subsistema físico no lineal "/1(T_l)
  "Subsistema físico no lineal "/2(T_s) -> Gain1/1
  "Subsistema físico no lineal "/1(theta_m) -> Gain/1
  Tº_amb/1 -> "Subsistema físico no lineal "/6(Tº_amb)
  "Subsistema físico no lineal "/4(i_bs) -> Gain3/1
  "Subsistema físico no lineal "/5(i_cs) -> Gain4/1
  "Subsistema físico no lineal "/3(i_as) -> Gain2/1
  Gain2/1 -> TD_PARK/1(fas), Mux/1
  Gain3/1 -> TD_PARK/2(fbs), Mux/2
  Gain4/1 -> TD_PARK/3(fcs), Mux/3
  Mux/1 -> i_abcs/1
  Gain/1 -> Gain8/1, theta_m/1
  "Subsistema físico no lineal "/6(omega_m) -> omega_m/1, Product1/1, Product/1  "omega_m"
  Gain1/1 -> T_s/1
  Gain8/1 -> "Subsistema físico no lineal "/5(theta_r), TI_PARK/4(theta_r), TD_PARK/4(theta_r)  "theta_r"
  TD_PARK/1(fqs) -> Mux1/1, Product/2  "i_qs^r"
  Product/1 -> Gain9/1
  Gain9/1 -> Gain10/1
  Gain11/1 -> mux/2, TI_PARK/2(fds)
  Gain10/1 -> Gain11/1
  Constant/1 -> TI_PARK/3(f0s), mux/3
  Inversor: Modulador de tensión/1(v_as) -> "Subsistema físico no lineal "/2(v_as)
  Inversor: Modulador de tensión/2(v_bs) -> "Subsistema físico no lineal "/3(v_bs)
  Inversor: Modulador de tensión/3(v_cs) -> "Subsistema físico no lineal "/4(v_cs)
  TI_PARK/1(fas) -> Mux2/1, Inversor: Modulador de tensión/1(v_as*)
  TI_PARK/2(fbs) -> Mux2/2, Inversor: Modulador de tensión/2(v_bs*)
  TI_PARK/3(fcs) -> Mux2/3, Inversor: Modulador de tensión/3(v_cs*)
  TD_PARK/2(fds) -> Mux1/2, Product1/2  "i_ds^r"
  TD_PARK/3(f0s) -> Mux1/3  "i_0s"
  v_qs/1 -> Sum/1
  Sum/1 -> mux/1, TI_PARK/1(fqs)
  Product1/1 -> Gain5/1
  Gain5/1 -> Gain6/1
  Gain6/1 -> Sum/2
  Mux1/1 -> iqd0s/1
  mux/1 -> v_qd0/1
  Mux2/1 -> v_abc/1
  "Subsistema físico no lineal "/7(T_m) -> T_m/1

== system main/Sistema linealizado por retroalimentación no lineal2 ==
  note: Entrada de perturbación
  note: Entrada de manipulación
  note: Entrada de perturbación
  note: Controlador
  note: Salida medida
  note: Controlador
  note: Sensores
  note: Salida medida
  note: Salidas medidas
  note: Salida no medida.
  note: Controlador
  T_l : Inport
  Tº_amb : Inport  Port=2
  v_qs : Inport  Port=3
  Constant : Constant  Value=0
  Gain{,1..4} (5 alike) : Gain
  Gain10 : Gain  Gain=L_q
  Gain11 : Gain  Gain=-1
  Gain5 : Gain  Gain=P_p
  Gain6 : Gain  Gain=L_d
  Gain8 : Gain  Gain=P_p
  Gain9 : Gain  Gain=P_p
  Inversor: Modulador de tensión : Subsystem
  Mux : Mux  Inputs=3
  Mux1 : Mux  Inputs=3
  Mux2 : Mux  Inputs=3
  Product : Product
  Product1 : Product
  "Subsistema físico no lineal " : Subsystem
      settings: PortSchema="{\"entries\":[{\"content\":{\"sides\":[{\"content\":{\"connectorIds\":[\"In1\",\"In2\",\"In3\",\"In4\",\"In5\",\"In6\"]},\"type\":\"ConnectorPlacement.EquallySpacedRectSide\",\"uuid\":\"df16c937-5b0d-437b-9581-4e7e4443d731\"},{\"content\":{\"connectorIds\":[\"Out1\",\"Out2\",\"Out3\",\"Out4\",\"Out5\"],\"side\":\"RIGHT\"},\"type\":\"ConnectorPlacement.EquallySpacedRectSide\",\"uuid\":\"58799b56-1bb2-4861-ad63-3fa3f8181ad5\"},{\"content\":{\"connectorIds\":[\"Out6\",\"Out7\"],\"side\":\"TOP\"},\"type\":\"ConnectorPlacement.EquallySpacedRectSide\",\"uuid\":\"9d658df7-49d2-4fa1-a84c-b158d9dac98e\"}]},\"type\":\"ConnectorPlacement.EquallySpacedConnector\",\"uuid\":\"4e139d46-6a94-417e-9cad-9c9676c83a39\"}],\"packageUris\":[\"http://schema.mathworks.com/mf0/Connector/R2020b\"],\"version\":\"1.0\"}"
  Sum : Sum  Inputs=|++
  TD_PARK : MATLAB Function  TreatAsAtomicUnit=on
  TI_PARK : MATLAB Function  TreatAsAtomicUnit=on
  mux : Mux  Inputs=3
  i_abcs : Outport
  theta_m : Outport  Port=2
  omega_m : Outport  Port=3
  T_s : Outport  Port=4
  iqd0s : Outport  Port=5
  v_qd0 : Outport  Port=6
  v_abc : Outport  Port=7
  T_m : Outport  Port=8
  wires:
  T_l/1 -> "Subsistema físico no lineal "/1(T_l)
  "Subsistema físico no lineal "/2(T_s) -> Gain1/1
  "Subsistema físico no lineal "/1(theta_m) -> Gain/1
  Tº_amb/1 -> "Subsistema físico no lineal "/6(Tº_amb)
  "Subsistema físico no lineal "/4(i_bs) -> Gain3/1
  "Subsistema físico no lineal "/5(i_cs) -> Gain4/1
  "Subsistema físico no lineal "/3(i_as) -> Gain2/1
  Gain2/1 -> TD_PARK/1(fas), Mux/1
  Gain3/1 -> TD_PARK/2(fbs), Mux/2
  Gain4/1 -> TD_PARK/3(fcs), Mux/3
  Mux/1 -> i_abcs/1
  Gain/1 -> Gain8/1, theta_m/1
  "Subsistema físico no lineal "/6(omega_m) -> omega_m/1, Product1/1, Product/1  "omega_m"
  Gain1/1 -> T_s/1
  Gain8/1 -> "Subsistema físico no lineal "/5(theta_r), TI_PARK/4(theta_r), TD_PARK/4(theta_r)  "theta_r"
  TD_PARK/1(fqs) -> Mux1/1, Product/2  "i_qs^r"
  Product/1 -> Gain9/1
  Gain9/1 -> Gain10/1
  Gain11/1 -> mux/2, TI_PARK/2(fds)
  Gain10/1 -> Gain11/1
  Constant/1 -> TI_PARK/3(f0s), mux/3
  Inversor: Modulador de tensión/1(v_as) -> "Subsistema físico no lineal "/2(v_as)
  Inversor: Modulador de tensión/2(v_bs) -> "Subsistema físico no lineal "/3(v_bs)
  Inversor: Modulador de tensión/3(v_cs) -> "Subsistema físico no lineal "/4(v_cs)
  TI_PARK/1(fas) -> Mux2/1, Inversor: Modulador de tensión/1(v_as*)
  TI_PARK/2(fbs) -> Mux2/2, Inversor: Modulador de tensión/2(v_bs*)
  TI_PARK/3(fcs) -> Mux2/3, Inversor: Modulador de tensión/3(v_cs*)
  TD_PARK/2(fds) -> Mux1/2, Product1/2  "i_ds^r"
  TD_PARK/3(f0s) -> Mux1/3  "i_0s"
  v_qs/1 -> Sum/1
  Sum/1 -> mux/1, TI_PARK/1(fqs)
  Product1/1 -> Gain5/1
  Gain5/1 -> Gain6/1
  Gain6/1 -> Sum/2
  Mux1/1 -> iqd0s/1
  mux/1 -> v_qd0/1
  Mux2/1 -> v_abc/1
  "Subsistema físico no lineal "/7(T_m) -> T_m/1

== system main/Sistema linealizado por retroalimentación no lineal3 ==
  note: Entrada de perturbación
  note: Entrada de manipulación
  note: Entrada de perturbación
  note: Controlador
  note: Salida medida
  note: Controlador
  note: Sensores
  note: Salida medida
  note: Salidas medidas
  note: Salida no medida.
  note: Controlador
  T_l : Inport
  Tº_amb : Inport  Port=2
  v_qs : Inport  Port=3
  Constant : Constant  Value=0
  Gain{,1..4} (5 alike) : Gain
  Gain10 : Gain  Gain=L_q
  Gain11 : Gain  Gain=-1
  Gain5 : Gain  Gain=P_p
  Gain6 : Gain  Gain=L_d
  Gain8 : Gain  Gain=P_p
  Gain9 : Gain  Gain=P_p
  Inversor: Modulador de tensión : Subsystem
  Mux : Mux  Inputs=3
  Mux1 : Mux  Inputs=3
  Mux2 : Mux  Inputs=3
  Product : Product
  Product1 : Product
  "Subsistema físico no lineal " : Subsystem
      settings: PortSchema="{\"entries\":[{\"content\":{\"sides\":[{\"content\":{\"connectorIds\":[\"In1\",\"In2\",\"In3\",\"In4\",\"In5\",\"In6\"]},\"type\":\"ConnectorPlacement.EquallySpacedRectSide\",\"uuid\":\"df16c937-5b0d-437b-9581-4e7e4443d731\"},{\"content\":{\"connectorIds\":[\"Out1\",\"Out2\",\"Out3\",\"Out4\",\"Out5\"],\"side\":\"RIGHT\"},\"type\":\"ConnectorPlacement.EquallySpacedRectSide\",\"uuid\":\"58799b56-1bb2-4861-ad63-3fa3f8181ad5\"},{\"content\":{\"connectorIds\":[\"Out6\",\"Out7\"],\"side\":\"TOP\"},\"type\":\"ConnectorPlacement.EquallySpacedRectSide\",\"uuid\":\"9d658df7-49d2-4fa1-a84c-b158d9dac98e\"}]},\"type\":\"ConnectorPlacement.EquallySpacedConnector\",\"uuid\":\"4e139d46-6a94-417e-9cad-9c9676c83a39\"}],\"packageUris\":[\"http://schema.mathworks.com/mf0/Connector/R2020b\"],\"version\":\"1.0\"}"
  Sum : Sum  Inputs=|++
  TD_PARK : MATLAB Function  TreatAsAtomicUnit=on
  TI_PARK : MATLAB Function  TreatAsAtomicUnit=on
  mux : Mux  Inputs=3
  i_abcs : Outport
  theta_m : Outport  Port=2
  omega_m : Outport  Port=3
  T_s : Outport  Port=4
  iqd0s : Outport  Port=5
  v_qd0 : Outport  Port=6
  v_abc : Outport  Port=7
  T_m : Outport  Port=8
  wires:
  T_l/1 -> "Subsistema físico no lineal "/1(T_l)
  "Subsistema físico no lineal "/2(T_s) -> Gain1/1
  "Subsistema físico no lineal "/1(theta_m) -> Gain/1
  Tº_amb/1 -> "Subsistema físico no lineal "/6(Tº_amb)
  "Subsistema físico no lineal "/4(i_bs) -> Gain3/1
  "Subsistema físico no lineal "/5(i_cs) -> Gain4/1
  "Subsistema físico no lineal "/3(i_as) -> Gain2/1
  Gain2/1 -> TD_PARK/1(fas), Mux/1
  Gain3/1 -> TD_PARK/2(fbs), Mux/2
  Gain4/1 -> TD_PARK/3(fcs), Mux/3
  Mux/1 -> i_abcs/1
  Gain/1 -> Gain8/1, theta_m/1
  "Subsistema físico no lineal "/6(omega_m) -> omega_m/1, Product1/1, Product/1  "omega_m"
  Gain1/1 -> T_s/1
  Gain8/1 -> "Subsistema físico no lineal "/5(theta_r), TI_PARK/4(theta_r), TD_PARK/4(theta_r)  "theta_r"
  TD_PARK/1(fqs) -> Mux1/1, Product/2  "i_qs^r"
  Product/1 -> Gain9/1
  Gain9/1 -> Gain10/1
  Gain11/1 -> mux/2, TI_PARK/2(fds)
  Gain10/1 -> Gain11/1
  Constant/1 -> TI_PARK/3(f0s), mux/3
  Inversor: Modulador de tensión/1(v_as) -> "Subsistema físico no lineal "/2(v_as)
  Inversor: Modulador de tensión/2(v_bs) -> "Subsistema físico no lineal "/3(v_bs)
  Inversor: Modulador de tensión/3(v_cs) -> "Subsistema físico no lineal "/4(v_cs)
  TI_PARK/1(fas) -> Mux2/1, Inversor: Modulador de tensión/1(v_as*)
  TI_PARK/2(fbs) -> Mux2/2, Inversor: Modulador de tensión/2(v_bs*)
  TI_PARK/3(fcs) -> Mux2/3, Inversor: Modulador de tensión/3(v_cs*)
  TD_PARK/2(fds) -> Mux1/2, Product1/2  "i_ds^r"
  TD_PARK/3(f0s) -> Mux1/3  "i_0s"
  v_qs/1 -> Sum/1
  Sum/1 -> mux/1, TI_PARK/1(fqs)
  Product1/1 -> Gain5/1
  Gain5/1 -> Gain6/1
  Gain6/1 -> Sum/2
  Mux1/1 -> iqd0s/1
  mux/1 -> v_qd0/1
  Mux2/1 -> v_abc/1
  "Subsistema físico no lineal "/7(T_m) -> T_m/1
